simulink model "bd_inv_cont_1tank"  (R2021b)
settings: Solver=VariableStepAuto  StartTime=0.0  StopTime=200  RelTol=1e-3
libraries: dspsrcs4 x1
settings Model: Creator=billtubbs  LastModifiedBy=billtubbs

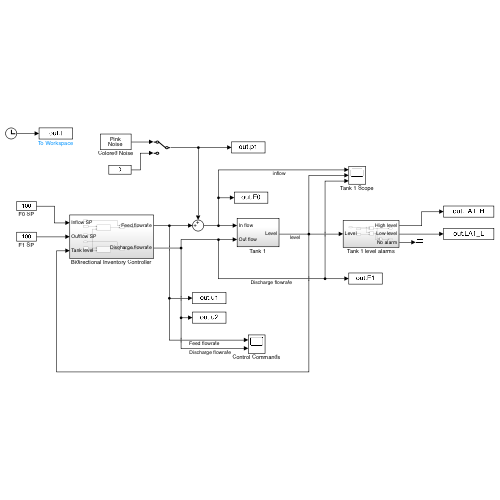
[thumbnail: Simulink's stored preview of the top-level diagram]
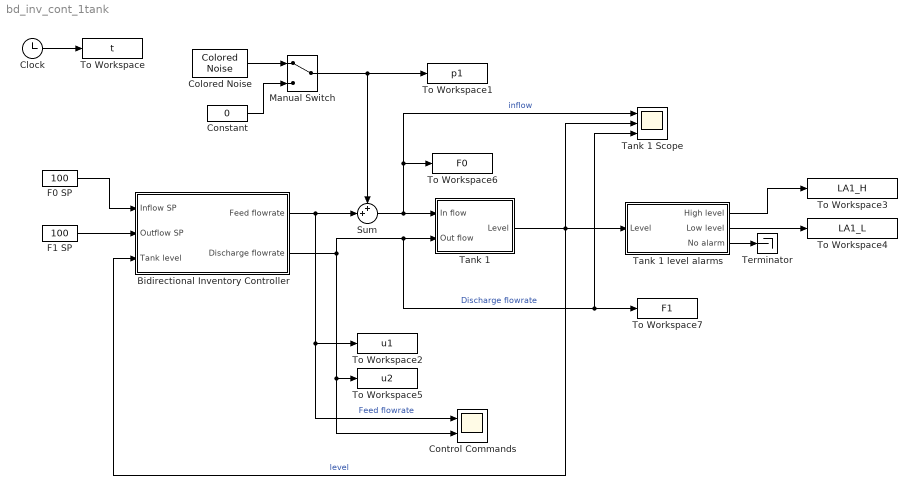
== system bd_inv_cont_1tank ==
  Bidirectional Inventory Controller : Subsystem
  Clock : Clock
  Colored Noise : dspsrcs4/Colored Noise  Color=pink  InverseFrequencyPower=1  BoundedOutput=off  NumChannels=1  OutputDataType=double  SamplesPerFrame=1  SampleTime=1  RandomStream=mt19937ar with seed  Seed=67  SimulateUsing=Interpreted execution
      settings: SourceProductBaseCode=DS
  Constant : Constant  Value=0
  Control Commands : Scope  NumInputPorts=2
  F0 SP : Constant  Value=100
  F1 SP : Constant  Value=100
  Manual Switch : ManualSwitch
  Sum : Sum  Inputs=++|
  Tank 1 : Subsystem
  Tank 1 Scope : Scope  NumInputPorts=3
  Tank 1 level alarms : Subsystem
  Terminator : Terminator
  To Workspace : ToWorkspace  VariableName=t  SaveFormat=Timeseries  SampleTime=-1
  To Workspace1 : ToWorkspace  VariableName=p1  SaveFormat=Timeseries  SampleTime=-1
  To Workspace2 : ToWorkspace  VariableName=u1  SaveFormat=Timeseries  SampleTime=-1
  To Workspace3 : ToWorkspace  VariableName=LA1_H  SaveFormat=Timeseries  SampleTime=-1
  To Workspace4 : ToWorkspace  VariableName=LA1_L  SaveFormat=Timeseries  SampleTime=-1
  To Workspace5 : ToWorkspace  VariableName=u2  SaveFormat=Timeseries  SampleTime=-1
  To Workspace6 : ToWorkspace  VariableName=F0  SaveFormat=Timeseries  SampleTime=-1
  To Workspace7 : ToWorkspace  VariableName=F1  SaveFormat=Timeseries  SampleTime=-1
  wires:
  Clock/1 -> To Workspace/1
  Bidirectional Inventory Controller/2(Discharge flowrate) -> Control Commands/2, To Workspace5/1, Tank 1 Scope/3, To Workspace7/1, Tank 1/2(Out flow)  "Discharge flowrate"
  Tank 1 level alarms/3(No alarm) -> Terminator/1
  Sum/1 -> Tank 1/1(In flow), Tank 1 Scope/1, To Workspace6/1  "inflow"
  Manual Switch/1 -> Sum/1, To Workspace1/1
  Tank 1 level alarms/1(High level) -> To Workspace3/1
  Tank 1 level alarms/2(Low level) -> To Workspace4/1
  Bidirectional Inventory Controller/1(Feed flowrate) -> To Workspace2/1, Control Commands/1, Sum/2  "Feed flowrate"
  Tank 1/1(Level) -> Bidirectional Inventory Controller/3(Tank level), Tank 1 Scope/2, Tank 1 level alarms/1(Level)  "level"
  Constant/1 -> Manual Switch/2
  Colored Noise/1 -> Manual Switch/1
  F0 SP/1 -> Bidirectional Inventory Controller/1(Inflow SP)
  F1 SP/1 -> Bidirectional Inventory Controller/2(Outflow SP)

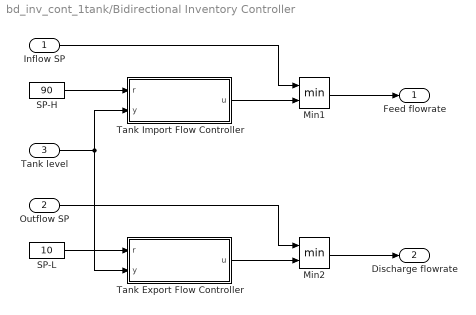
== system bd_inv_cont_1tank/Bidirectional Inventory Controller ==
  Inflow SP : Inport
  Outflow SP : Inport  Port=2
  Tank level : Inport  Port=3
  Min1 : MinMax  Inputs=2
  Min2 : MinMax  Inputs=2
  SP-H : Constant  Value=90
  SP-L : Constant  Value=10
  Tank Export Flow Controller : Subsystem
  Tank Import Flow Controller : Subsystem
  Feed flowrate : Outport
  Discharge flowrate : Outport  Port=2
  wires:
  Tank Import Flow Controller/1(u) -> Min1/2
  Outflow SP/1 -> Min2/1
  Tank Export Flow Controller/1(u) -> Min2/2
  Tank level/1 -> Tank Export Flow Controller/2(y), Tank Import Flow Controller/2(y)
  SP-H/1 -> Tank Import Flow Controller/1(r)
  SP-L/1 -> Tank Export Flow Controller/1(r)
  Inflow SP/1 -> Min1/1
  Min1/1 -> Feed flowrate/1
  Min2/1 -> Discharge flowrate/1

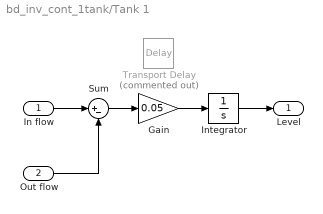
== system bd_inv_cont_1tank/Tank 1 ==
  In flow : Inport
  Out flow : Inport  Port=2
  Gain : Gain  Gain=0.05
  Integrator : Integrator
  Sum : Sum  Inputs=|+-
  Transport Delay : TransportDelay  Commented=on  DelayTime=0
  Level : Outport  InitialOutput=0
  wires:
  Sum/1 -> Gain/1
  Integrator/1 -> Level/1
  In flow/1 -> Sum/1
  Out flow/1 -> Sum/2
  Gain/1 -> Integrator/1

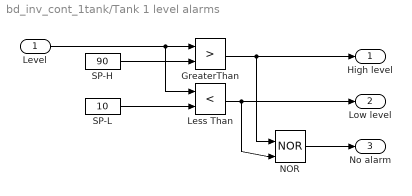
== system bd_inv_cont_1tank/Tank 1 level alarms ==
  Level : Inport
  GreaterThan : RelationalOperator  Operator=>  OutDataTypeStr=boolean  RndMeth=Simplest
  Less Than : RelationalOperator  Operator=<  OutDataTypeStr=boolean  RndMeth=Simplest
  NOR : Logic  Operator=NOR  IconShape=distinctive  AllPortsSameDT=off  OutDataTypeStr=boolean
  SP-H : Constant  Value=90
  SP-L : Constant  Value=10
  High level : Outport
  Low level : Outport  Port=2
  No alarm : Outport  Port=3
  wires:
  Level/1 -> Less Than/1, GreaterThan/1
  SP-L/1 -> Less Than/2
  GreaterThan/1 -> High level/1, NOR/1
  SP-H/1 -> GreaterThan/2
  Less Than/1 -> NOR/2, Low level/1
  NOR/1 -> No alarm/1

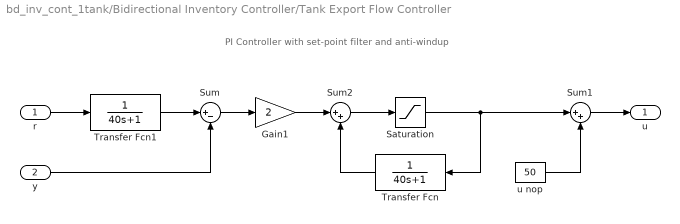
== system bd_inv_cont_1tank/Bidirectional Inventory Controller/Tank Export Flow Controller ==
  note: PI Controller with set-point filter and anti-windup
  r : Inport
  y : Inport  Port=2
  Gain1 : Gain  Gain=2
  Saturation : Saturate  UpperLimit=50  LowerLimit=-50
  Sum : Sum  Inputs=|+-
  Sum1 : Sum  Inputs=|++
  Sum2 : Sum  Inputs=|++
  Transfer Fcn : TransferFcn  Denominator=[40 1]
  Transfer Fcn1 : TransferFcn  Denominator=[40 1]
  u nop : Constant  Value=50
  u : Outport
  wires:
  r/1 -> Transfer Fcn1/1
  Sum1/1 -> u/1
  Saturation/1 -> Transfer Fcn/1, Sum1/1
  u nop/1 -> Sum1/2
  Sum/1 -> Gain1/1
  y/1 -> Sum/2
  Transfer Fcn/1 -> Sum2/2
  Sum2/1 -> Saturation/1
  Gain1/1 -> Sum2/1
  Transfer Fcn1/1 -> Sum/1

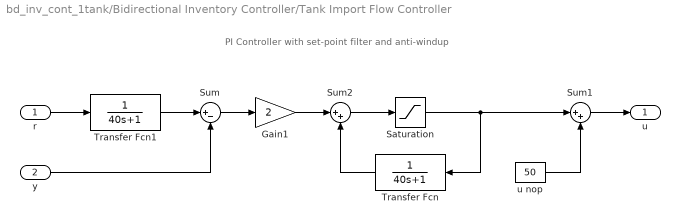
== system bd_inv_cont_1tank/Bidirectional Inventory Controller/Tank Import Flow Controller ==
  note: PI Controller with set-point filter and anti-windup
  r : Inport
  y : Inport  Port=2
  Gain1 : Gain  Gain=2
  Saturation : Saturate  UpperLimit=50  LowerLimit=-50
  Sum : Sum  Inputs=|+-
  Sum1 : Sum  Inputs=|++
  Sum2 : Sum  Inputs=|++
  Transfer Fcn : TransferFcn  Denominator=[40 1]
  Transfer Fcn1 : TransferFcn  Denominator=[40 1]
  u nop : Constant  Value=50
  u : Outport
  wires:
  r/1 -> Transfer Fcn1/1
  Sum1/1 -> u/1
  Saturation/1 -> Transfer Fcn/1, Sum1/1
  u nop/1 -> Sum1/2
  Sum/1 -> Gain1/1
  y/1 -> Sum/2
  Transfer Fcn/1 -> Sum2/2
  Sum2/1 -> Saturation/1
  Gain1/1 -> Sum2/1
  Transfer Fcn1/1 -> Sum/1
